simulink model "lab_otu_pid_mod"  (R2023a)
settings: Solver=VariableStepAuto  StartTime=0.0  StopTime=10  RelTol=1e-3
settings Model: Creator=gnomy  LastModifiedBy=gnomy

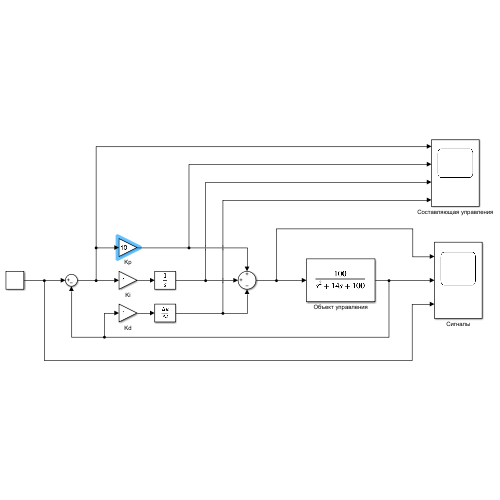
[thumbnail: Simulink's stored preview of the top-level diagram]
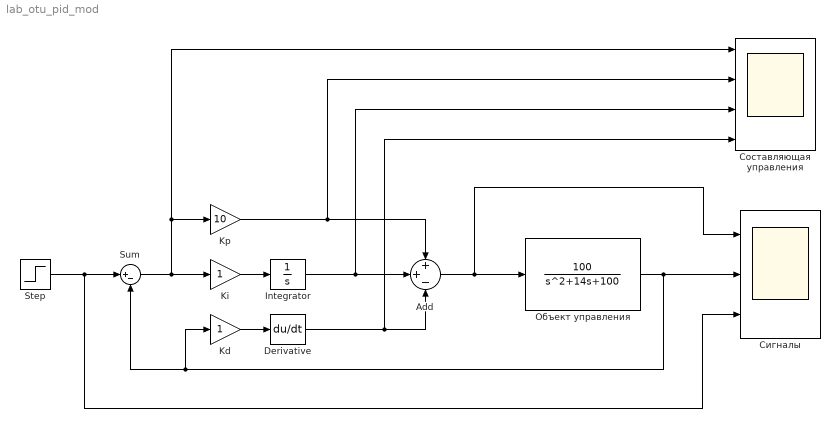
== system lab_otu_pid_mod ==
  Add : Sum  Inputs=++-
  Derivative : Derivative
  Integrator : Integrator
  Kd : Gain
  Ki : Gain
  Kp : Gain  Gain=10
  Step : Step  SampleTime=0
  Sum : Sum  Inputs=|+-
  Объект управления : TransferFcn  Numerator=[100]  Denominator=[1 14 100]
  Сигналы : Scope  NumInputPorts=3
  Составляющая управления : Scope  NumInputPorts=4
  wires:
  Ki/1 -> Integrator/1
  Kd/1 -> Derivative/1
  Kp/1 -> Составляющая управления/2, Add/1
  Integrator/1 -> Составляющая управления/3, Add/2
  Derivative/1 -> Составляющая управления/4, Add/3
  Sum/1 -> Kp/1, Составляющая управления/1, Ki/1
  Add/1 -> Сигналы/1, Объект управления/1
  Step/1 -> Сигналы/3, Sum/1
  Объект управления/1 -> Kd/1, Sum/2, Сигналы/2
